simulink model "MIMO_FourBlockModel"  (R2025b)
settings: Solver=VariableStepAuto  StartTime=0.0  StopTime=10.0  RelTol=1e-3
libraries: Drone_MIMO_Simple_Model x1
settings Model: Creator=Alek  LastModifiedBy=Alek

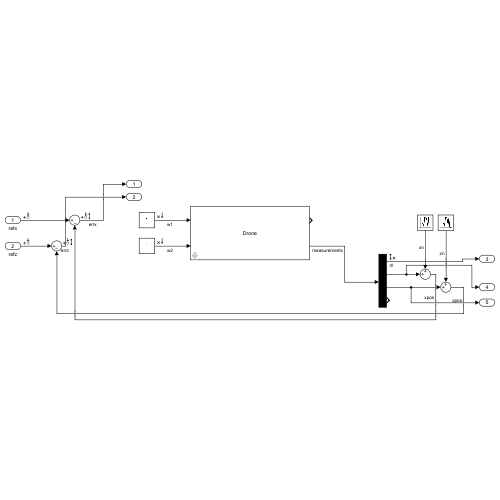
[thumbnail: Simulink's stored preview of the top-level diagram]
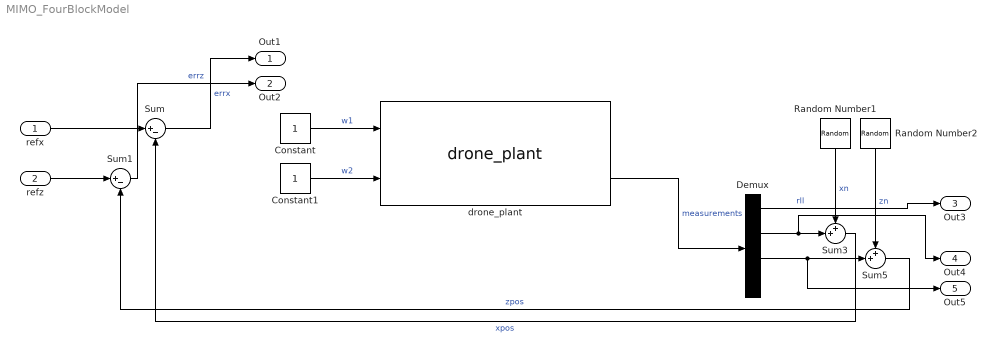
== system MIMO_FourBlockModel ==
  refx : Inport
  refz : Inport  Port=2
  Constant : Constant
  Constant1 : Constant
  Demux : Demux
  Random Number1 : RandomNumber  SampleTime=0.001
  Random Number2 : RandomNumber  SampleTime=0.001
  Sum : Sum  Inputs=|+-
  Sum1 : Sum  Inputs=|+-
  Sum3 : Sum  Inputs=++|
  Sum5 : Sum  Inputs=++|
  drone_plant : Drone_MIMO_Simple_Model/drone_plant  kf=1e-5  m=0.5  l=1e-2  Irod=6.6666e-5
      settings: SourceProductName=DroneLibrary
  Out1 : Outport
  Out2 : Outport  Port=2
  Out3 : Outport  Port=3
  Out4 : Outport  Port=4
  Out5 : Outport  Port=5
  wires:
  Constant/1 -> drone_plant/1  "w1"
  Constant1/1 -> drone_plant/2  "w2"
  drone_plant/2 -> Demux/1  "measurements"
  refz/1 -> Sum1/1
  refx/1 -> Sum/1
  Sum/1 -> Out1/1  "errx"
  Sum1/1 -> Out2/1  "errz"
  Demux/1 -> Out3/1  "rll"
  Demux/2 -> Out4/1, Sum3/2
  Demux/3 -> Out5/1, Sum5/2
  Random Number1/1 -> Sum3/1  "xn"
  Random Number2/1 -> Sum5/1  "zn"
  Sum3/1 -> Sum/2  "xpos"
  Sum5/1 -> Sum1/2  "zpos"
